simulink model "SIR_model"  (R2023a)
settings: Solver=VariableStepAuto  StartTime=0.0  StopTime=30  RelTol=1e-3
values from neighbouring files (symbols this model uses):
  b = 1.2    [parameters_covid.mat]
  g = 0.1    [parameters_covid.mat]
  N = 7500000    [parameters_covid.mat]
settings Model: Creator=mluser  LastModifiedBy=mluser

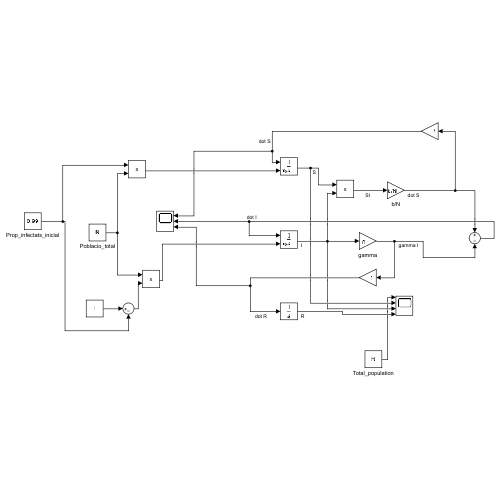
[thumbnail: Simulink's stored preview of the top-level diagram]
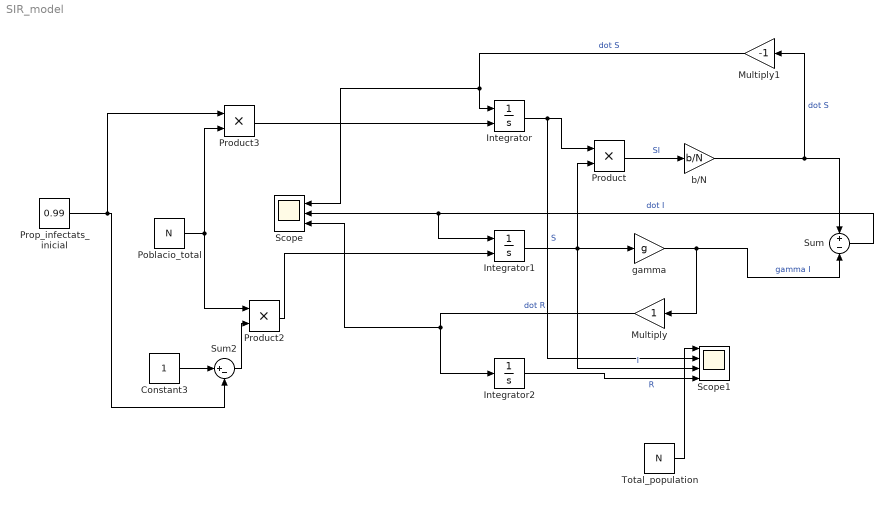
== system SIR_model ==
  Constant3 : Constant
  Integrator : Integrator  InitialConditionSource=external  InitialCondition=N
  Integrator1 : Integrator  InitialConditionSource=external
  Integrator2 : Integrator
  Multiply : Gain
  Multiply1 : Gain  Gain=-1
  Poblacio_total : Constant  Value=N
  Product : Product
  Product2 : Product
  Product3 : Product
  Prop_infectats_inicial : Constant  Value=0.99
  Scope : Scope  NumInputPorts=3
  Scope1 : Scope  NumInputPorts=4
  Sum : Sum  Inputs=+-
  Sum2 : Sum  Inputs=|+-
  Total_population : Constant  Value=N
  b/N : Gain  Gain=b/N
  gamma : Gain  Gain=g
  wires:
  Integrator/1 -> Product/1, Scope1/2  "S"
  Product/1 -> b/N/1  "SI"
  gamma/1 -> Multiply/1, Sum/2  "gamma I"
  Sum/1 -> Integrator1/1, Scope/2  "dot I"
  Multiply/1 -> Scope/3, Integrator2/1  "dot R"
  Integrator2/1 -> Scope1/4  "R"
  b/N/1 -> Multiply1/1, Sum/1  "dot S"
  Multiply1/1 -> Scope/1, Integrator/1  "dot S"
  Integrator1/1 -> gamma/1, Scope1/3, Product/2  "I"
  Prop_infectats_inicial/1 -> Product3/1, Sum2/2
  Sum2/1 -> Product2/2
  Constant3/1 -> Sum2/1
  Product3/1 -> Integrator/2
  Poblacio_total/1 -> Product2/1, Product3/2
  Product2/1 -> Integrator1/2
  Total_population/1 -> Scope1/1
